simulink model "pid_model_selector_motorlibreria"  (R2019b)
settings: Solver=FixedStepAuto  StartTime=0  StopTime=0.02  FixedStep=1e-7  RelTol=1e-3
values from neighbouring files (symbols this model uses):
  duty_input_voltage_100 = 1    [pid_values_motorlibreria.m]    (also in pid_values_motorlibreria_OperationPointA.m; pid_values_motorlibreria_OperationPointB.m; pid_values_motorlibreria_OperationPointC.m)
  Kb = 0    [pid_values_motorlibreria.m]    (also in pid_values_motorlibreria_OperationPointA.m = 0.00333333333333; pid_values_motorlibreria_OperationPointB.m = 0.00333333333333; pid_values_motorlibreria_OperationPointC.m = 0.00333333333333)
  Kd = 0    [pid_values_motorlibreria.m]    (also in pid_values_motorlibreria_OperationPointA.m; pid_values_motorlibreria_OperationPointB.m; pid_values_motorlibreria_OperationPointC.m)
  Ki = 0    [pid_values_motorlibreria.m]    (also in pid_values_motorlibreria_OperationPointA.m = 300; pid_values_motorlibreria_OperationPointB.m = 300; pid_values_motorlibreria_OperationPointC.m = 300)
  Kp = 1    [pid_values_motorlibreria.m]    (also in pid_values_motorlibreria_OperationPointA.m = 10; pid_values_motorlibreria_OperationPointB.m = 10; pid_values_motorlibreria_OperationPointC.m = 10)
  max_speed = 9500    [pid_values_motorlibreria.m]    (also in pid_values_motorlibreria_OperationPointA.m; pid_values_motorlibreria_OperationPointB.m; pid_values_motorlibreria_OperationPointC.m)
  motor_load = 251.26    [pid_values_motorlibreria.m]    (also in pid_values_motorlibreria_OperationPointA.m = -251.26; pid_values_motorlibreria_OperationPointB.m = -167.8; pid_values_motorlibreria_OperationPointC.m = -100.5)
  out_max = 1    [pid_values_motorlibreria.m]    (also in pid_values_motorlibreria_OperationPointA.m; pid_values_motorlibreria_OperationPointB.m; pid_values_motorlibreria_OperationPointC.m)
  out_min = -1    [pid_values_motorlibreria.m]    (also in pid_values_motorlibreria_OperationPointA.m; pid_values_motorlibreria_OperationPointB.m; pid_values_motorlibreria_OperationPointC.m)
  rads2rpm = 60/2/pi    (= 9.54929658551)    [pid_values_motorlibreria_OperationPointA.m]    (also in pid_values_motorlibreria_OperationPointB.m; pid_values_motorlibreria_OperationPointC.m)
  rotor_inertia = 536    [pid_values_motorlibreria.m]    (also in pid_values_motorlibreria_OperationPointA.m; pid_values_motorlibreria_OperationPointB.m; pid_values_motorlibreria_OperationPointC.m)
  speed_command = 3800    [pid_values_motorlibreria_OperationPointA.m]    (also in pid_values_motorlibreria_OperationPointB.m = 5690; pid_values_motorlibreria_OperationPointC.m = 9500)
undefined symbols (not defined in the file or in its folder): sigbuilder_block
libraries: fl_lib x10, nesl_utility x7, powerlib_meascontrol x4, ee_lib x3
settings Model: Creator=B00417  LastModifiedBy=B00417
settings SolverCC: ZeroCrossAlgorithm=Adaptive  AlgebraicLoopSolver=LineSearch
settings DebuggingCC: IgnoredZcDiagnostic=none

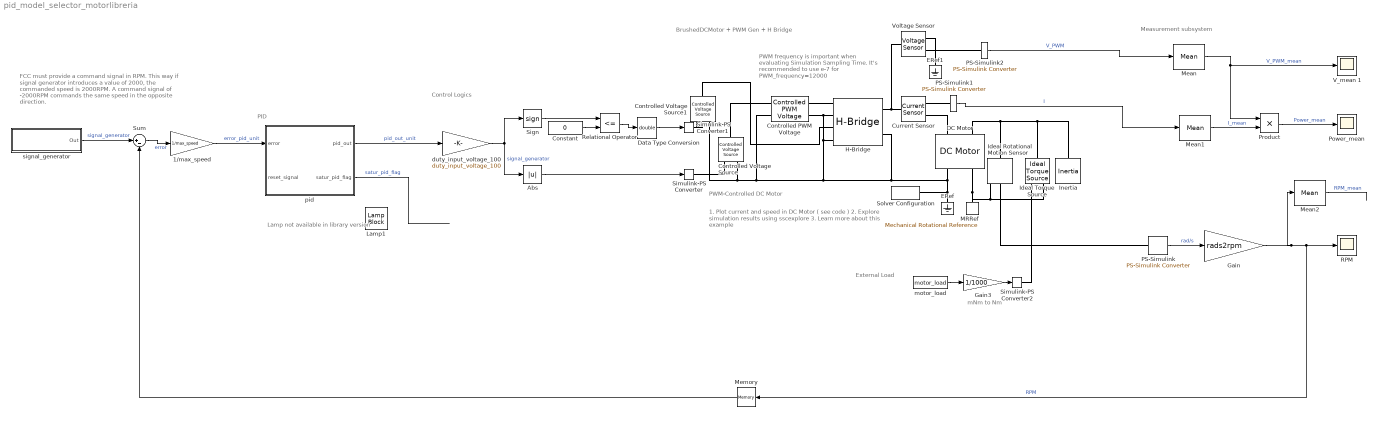
== system pid_model_selector_motorlibreria ==
  note: PWM frequency is important when evaluating Simulation Sampling Time.
      | It's recommended to use e-7 for PWM_frequency=12000
  note: External Load
  note: Control Logics
  note: FCC must provide a command signal in RPM. This way if signal generator introduces a value of 2000, the commanded speed is 2000RPM. A command signal of -2000RPM commands the same speed in the opposite direction.
  note: PID
  note: Lamp not available in library version
  note: Measurement subsystem
  note: BrushedDCMotor
      | + PWM Gen
      | + H Bridge
  note: mNm to Nm
  note: PWM-Controlled DC Motor
  note: 1. Plot current and speed in DC Motor ( see code )
      | 2. Explore simulation results using sscexplore
      | 3. Learn more about this example
  1/max_speed : Gain  Gain=1/max_speed
  Abs : Abs
  Constant : Constant  Value=0
  Controlled PWM Voltage : ee_lib/Integrated Circuits/Controlled PWM Voltage  F=PWM_frequency Hz  TD=PWM_delay s  pulse_width_offset=PWM_pulse_width_offset s  pulse_min=PWM_minimum_pulse_width s  Vmin=duty_input_voltage_0 V  Vmax=duty_input_voltage_100 V  Vm=V_duty_output V  pwm_or_av=1  event_type=1  sample_time=5e-6 s  u_min=0  u_max=1
      settings: SourceProductName=Simscape Electrical
  Controlled Voltage Source : fl_lib/Electrical/Electrical Sources/Controlled Voltage Source
  Controlled Voltage Source1 : fl_lib/Electrical/Electrical Sources/Controlled Voltage Source
  Current Sensor : fl_lib/Electrical/Electrical Sensors/Current Sensor
  DC Motor : ee_lib/Electromechanical/Brushed Motors/DC Motor  parameterization=2  Ra=3.38 Ohm  La=armature_inductance H  emf_or_torque=1  Kv=0.029 V/(rad/s)  Ki=6.876e-04 N*m/A  T_stall=stall_torque mN*m  w_max=no_load_speed rpm  w_rated=rated_speed rpm  P_rated=rated_load W  V_rated=rated_DC_V_supply V  J=rotor_inertia g*cm^2  lam_param=1  lam=rotor_damping N*m/(rad/s)  i_noload=728 mA  V_i_noload=20 V  speed0=0 rpm  alpha=3.93e-3 1/K  Tmeas=25 degC  thermal_mass=100 J/K  initial_temperature=25 degC
      settings: SourceProductName=Simscape Electrical
  Data Type Conversion : DataTypeConversion  OutMin=[0]  OutMax=[1]  OutDataTypeStr=double
  ERef : fl_lib/Electrical/Electrical Elements/Electrical Reference
  ERef1 : fl_lib/Electrical/Electrical Elements/Electrical Reference
  Gain : Gain  Gain=rads2rpm
  Gain3 : Gain  Gain=1/1000
  H-Bridge : ee_lib/Semiconductors & Converters/Converters/H-Bridge  supply_ports=ee.enum.supply_ports.hidesupply  Venable=V_enable V  Vmax=PWM_signal_amplitude V  Vreverse=REV_V V  Vbrake=BRK_V V  Vm=output_V V  pwm_or_av=ee.enum.pwm_or_av.pwm  regenerative_braking_mode=ee.enum.converters.regenerative_braking_mode.always_enabled  discontinuous=ee.enum.current_profile.continuous  freewheeling_mode=ee.enum.converters.freewheeling_mode.one_switch_one_diode  Ron=bridge_resistance Ohm  Don=diode_resistance Ohm  Goff=1e-6 S  Rload=3.38+0.1 Ohm  Lload=1e-5 H  F=4 kHz  thermal_mass=100 J/K  initial_temperature=298.15 K  Ron2=0.1 Ohm  Don2=0.05 Ohm  Tmeas=298.15 K  Tmeas2=398.15 K
      settings: SourceProductName=Simscape Electrical
  Ideal Rotational Motion Sensor : fl_lib/Mechanical/Mechanical Sensors/Ideal Rotational Motion Sensor  offset=0 deg
  Ideal Torque Source : fl_lib/Mechanical/Mechanical Sources/Ideal Torque Source
  Inertia : fl_lib/Mechanical/Rotational Elements/Inertia  inertia=motor_load_inertia kg*m^2  w_specify=off  w_priority=High  w=0 rad/s  w_nominal_specify=off  w_nominal_unit=rad/s  w_nominal_value=1  t_specify=off  t_priority=None  t=0 N*m  t_nominal_specify=off  t_nominal_unit=N*m  t_nominal_value=1
  Lamp1 : LampBlock
  MRRef : fl_lib/Mechanical/Rotational Elements/Mechanical Rotational Reference
  Mean : powerlib_meascontrol/Measurements/Mean  Freq=fundamental_frequency  Vinit=0  Ts=0
      settings: SourceProductName=Simscape Electrical
  Mean1 : powerlib_meascontrol/Measurements/Mean  Freq=fundamental_frequency  Vinit=0  Ts=0
      settings: SourceProductName=Simscape Electrical
  Mean2 : powerlib_meascontrol/Measurements/Mean  Freq=fundamental_frequency  Vinit=0  Ts=0
      settings: SourceProductName=Simscape Electrical
  Memory : Memory
  PS-Simulink : nesl_utility/PS-Simulink Converter  PhysicalDomain=network_engine_domain  SubClassName=ps_output  LeftPortType=input  RightPortType=output  PseudoPeriodic=off  Frequencies=[]  Unit=rpm  AffineConversion=off
  PS-Simulink1 : nesl_utility/PS-Simulink Converter  PhysicalDomain=network_engine_domain  SubClassName=ps_output  LeftPortType=input  RightPortType=output  PseudoPeriodic=off  Frequencies=[]  Unit=A  AffineConversion=off
  PS-Simulink2 : nesl_utility/PS-Simulink Converter  PhysicalDomain=network_engine_domain  SubClassName=ps_output  LeftPortType=input  RightPortType=output  PseudoPeriodic=off  Frequencies=[]  Unit=V  AffineConversion=off
  Power_mean : Scope
  Product : Product
  "RPM " : Scope
  Relational Operator : RelationalOperator  Operator=<=  OutDataTypeStr=boolean  RndMeth=Simplest
  Sign : Signum
  Simulink-PS Converter : nesl_utility/Simulink-PS Converter  PhysicalDomain=network_engine_domain  SubClassName=ps_input  LeftPortType=input  RightPortType=output  PseudoPeriodic=off  Frequencies=[]  NoiseDistribution=none  NoiseParameters=[]  Unit=1  AffineConversion=off  FilteringAndDerivatives=provide  SimscapeFilterOrder=1  InputFilterTimeConstant=0.001  UdotUserProvided=0
  Simulink-PS Converter1 : nesl_utility/Simulink-PS Converter  PhysicalDomain=network_engine_domain  SubClassName=ps_input  LeftPortType=input  RightPortType=output  PseudoPeriodic=off  Frequencies=[]  NoiseDistribution=none  NoiseParameters=[]  Unit=1  AffineConversion=off  FilteringAndDerivatives=provide  SimscapeFilterOrder=1  InputFilterTimeConstant=0.001  UdotUserProvided=0
  Simulink-PS Converter2 : nesl_utility/Simulink-PS Converter  PhysicalDomain=network_engine_domain  SubClassName=ps_input  LeftPortType=input  RightPortType=output  PseudoPeriodic=off  Frequencies=[]  NoiseDistribution=none  NoiseParameters=[]  Unit=1  AffineConversion=off  FilteringAndDerivatives=provide  SimscapeFilterOrder=1  InputFilterTimeConstant=0.001  UdotUserProvided=0
  Solver Configuration : nesl_utility/Solver Configuration  PhysicalDomain=network_engine_domain  SubClassName=solver  LeftPortType=input  RightPortType=generic  Tones=[]  Harmonics=[]  SimulateNoise=off  Profile=off  UseLocalSampling=off  EnableSwitchedLinearOptims=on  FrequencyDomain=off  UseCCode=off  RelTol=0.001  AbsTol=1e-06  MinStep=1e-09  ToWorkspace=off  RevertToSquareIcSolve=off  NumHomotopyIterations=100  PhasorMode=off  PhasorModeNumHarmonics=1  DoDC=off  ResidualTolerance=1e-9  UseLocalSolver=off  LocalSolverChoice=NE_BACKWARD_EULER_ADVANCER  LocalSolverSampleTime=1e-7  DoFixedCost=off  MaxNonlinIter=4  MaxModeIter=2  LinearAlgebra=auto  EquationFormulation=NE_TIME_EF  DelaysMemoryBudget=1024  AutomaticFiltering=on  FilteringTimeConstant=0.001  PartitionStorageMethod=AS_NEEDED  PartitionMemoryBudget=1024  PartitionMethod=FAST
  Sum : Sum  Inputs=|+-
  V_mean 1 : Scope
  Voltage Sensor : fl_lib/Electrical/Electrical Sensors/Voltage Sensor
  duty_input_voltage_100 : Gain  Gain=duty_input_voltage_100
  motor_load : Constant  Value=motor_load
  pid : Subsystem  mask{Kp=Kp, Ki=Ki, Kd=Kd, saturation_off=off, x_max=out_max, x_min=out_min, Ka=Kb}
      mask prompts: Kp "Kp Ganancia proporcional"; Ki "Ki Ganancia integral"; Kd "Kd Ganancia derivativa"; saturation_off "saturation off"; x_max "Salida máxima saturación"; x_min "salida minima satración"; Ka "Kb Ganancia Windup"
      mask DialogControl wind_up_container Prompt: saturation
      mask Display: disp("PID")
  "signal_generator " : Subsystem  mask{signal=Step, A=speed_command, f=10, Bias=0, Tstart=0, SlewRate=10000, SlewRate_Switch=off}
      mask prompts: A "Amplitude A"; f "Frequency f (Hz)"; Tstart "Start time for step Tstart (s)"; SlewRate "Maximum Slew Rate (1/s)"; SlewRate_Switch "On/Off"
      mask help:
      | Signal_generator
      |
      | Necesita:
      | Entender que es BIOS
      | Saw no funciona (Arreglar)
      |
      | Info:
      | Slew rate es el ratio de subida máximo que permite un generador, generalmente se mide en V/segundo. En este caso, un valor de 1 hace que la pendiente máxima sea 1.
      mask TypeOptions signal: Constant | Step | Sine | Step series | Saw | Builder
      mask Callback signal:
      | 1;
      | 2;
      | 3;
      | 4;
      | 5;
      mask Display: disp('signal_generator')
  wires:
  "signal_generator "/1(Out) -> Sum/1  "signal_generator"
  Sum/1 -> 1/max_speed/1  "error"
  1/max_speed/1 -> pid/1(error)  "error_pid_unit"
  pid/1(pid_out) -> duty_input_voltage_100/1  "pid_out_unit"
  pid/2(satur_pid_flag) -> ?  "satur_pid_flag"
  Mean1/1 -> Product/2  "I_mean"
  Mean/1 -> Product/1, V_mean 1/1  "V_PWM_mean"
  Constant/1 -> Relational Operator/2
  Sign/1 -> Relational Operator/1
  Relational Operator/1 -> Data Type Conversion/1
  PS-Simulink2/1 -> Mean/1  "V_PWM"
  PS-Simulink1/1 -> Mean1/1  "I"
  Abs/1 -> Simulink-PS Converter/1
  Product/1 -> Power_mean/1  "Power_mean"
  motor_load/1 -> Gain3/1
  PS-Simulink/1 -> Gain/1  "rad/s"
  Gain3/1 -> Simulink-PS Converter2/1
  Data Type Conversion/1 -> Simulink-PS Converter1/1
  duty_input_voltage_100/1 -> Abs/1, Sign/1  "signal_generator"
  Gain/1 -> Mean2/1, Memory/1, "RPM "/1  "RPM"
  Memory/1 -> Sum/2
  Mean2/1 -> ?  "RPM_mean"
  connections:
  H-Bridge/LConn2 -- Controlled PWM Voltage/RConn2 -- H-Bridge/RConn2 -- DC Motor/RConn1 -- Solver Configuration/RConn1 -- ERef/LConn1 -- Controlled Voltage Source1/RConn2 -- Controlled Voltage Source/RConn2 -- Controlled PWM Voltage/LConn2 -- H-Bridge/LConn4
  H-Bridge/RConn1 -- Voltage Sensor/LConn1 -- Current Sensor/LConn1
  MRRef/LConn1 -- Ideal Torque Source/RConn2 -- Ideal Rotational Motion Sensor/RConn1 -- DC Motor/RConn2
  Simulink-PS Converter/RConn1 -- Controlled Voltage Source/RConn1
  Current Sensor/RConn2 -- DC Motor/LConn1
  Simulink-PS Converter2/RConn1 -- Ideal Torque Source/RConn1
  Controlled Voltage Source1/LConn1 -- H-Bridge/LConn3
  Controlled Voltage Source/LConn1 -- Controlled PWM Voltage/LConn1
  Controlled PWM Voltage/RConn1 -- H-Bridge/LConn1
  Simulink-PS Converter1/RConn1 -- Controlled Voltage Source1/RConn1
  Current Sensor/RConn1 -- PS-Simulink1/LConn1
  Voltage Sensor/RConn1 -- PS-Simulink2/LConn1
  Ideal Rotational Motion Sensor/RConn2 -- PS-Simulink/LConn1
  DC Motor/LConn2 -- Ideal Rotational Motion Sensor/LConn1 -- Ideal Torque Source/LConn1 -- Inertia/LConn1
  Voltage Sensor/RConn2 -- ERef1/LConn1

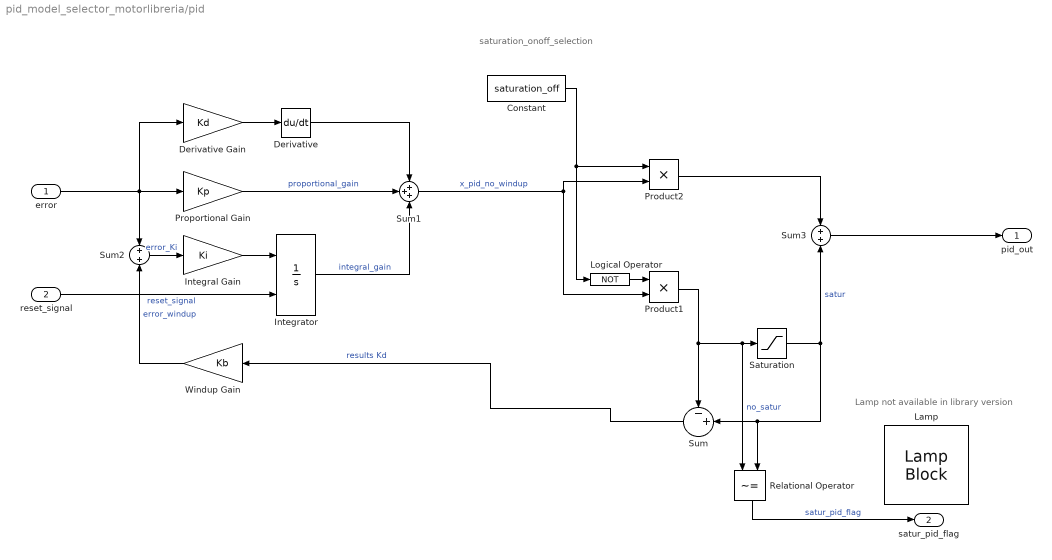
== system pid_model_selector_motorlibreria/pid ==
  note: Lamp not available in library version
  note: saturation_onoff_selection
  error : Inport
  reset_signal : Inport  Port=2
  Constant : Constant  Value=saturation_off
  Derivative : Derivative
  Derivative Gain : Gain  Gain=Kd
  Integral Gain : Gain  DisableCoverage=on  Gain=Ki
  Integrator : Integrator  ExternalReset=falling
  Lamp : LampBlock
  Logical Operator : Logic  Operator=NOT  AllPortsSameDT=off  OutDataTypeStr=boolean
  Product1 : Product
  Product2 : Product
  Proportional Gain : Gain  Gain=Kp
  Relational Operator : RelationalOperator  Operator=~=  OutDataTypeStr=boolean  RndMeth=Simplest
  Saturation : Saturate  UpperLimit=x_max  LowerLimit=x_min
  Sum : Sum  Inputs=-+|
  Sum1 : Sum  Inputs=+++
  Sum2 : Sum  Inputs=+|+
  Sum3 : Sum  Inputs=+|+
  Windup Gain : Gain  DisableCoverage=on  Gain=Kb
  pid_out : Outport
  satur_pid_flag : Outport  Port=2
  wires:
  Integrator/1 -> Sum1/3  "integral_gain"
  Integral Gain/1 -> Integrator/1
  error/1 -> Derivative Gain/1, Proportional Gain/1, Sum2/1
  Sum1/1 -> Product1/2, Product2/2  "x_pid_no_windup"
  Proportional Gain/1 -> Sum1/2  "proportional_gain"
  reset_signal/1 -> Integrator/2  "reset_signal"
  Saturation/1 -> Sum3/2, Relational Operator/2, Sum/2  "satur"
  Sum2/1 -> Integral Gain/1  "error_Ki"
  Sum/1 -> Windup Gain/1  "results Kd"
  Windup Gain/1 -> Sum2/2  "error_windup"
  Derivative Gain/1 -> Derivative/1
  Derivative/1 -> Sum1/1
  Relational Operator/1 -> satur_pid_flag/1  "satur_pid_flag"
  Sum3/1 -> pid_out/1
  Product2/1 -> Sum3/1
  Product1/1 -> Saturation/1, Relational Operator/1, Sum/1  "no_satur"
  Constant/1 -> Product2/1, Logical Operator/1
  Logical Operator/1 -> Product1/1

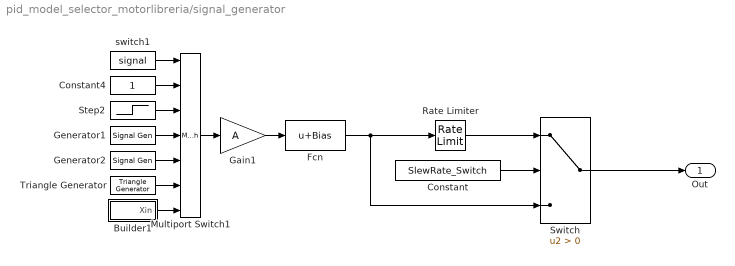
== system pid_model_selector_motorlibreria/signal_generator  ==
  Builder1 : Subsystem  Tag=STV Subsys  LoadFcn=sigbuilder_block('load');  StartFcn=sigbuilder_block('start');  StopFcn=sigbuilder_block('stop');  ClipboardFcn=sigbuilder_block('clipboard');  mask(Sigbuilder block){tuvar=[0:10]}
      mask help: Simulink:masks:SigbuilderBlock_MD
      mask init:
      | if ~strcmp(get_param(bdroot(gcbh),'SimulationStatus'),'stopped') tuvar = sigbuilder_block('maskInit'); end
      settings: CopyFcn=sigbuilder_block('copy');  DeleteFcn=sigbuilder_block('delete');  ModelCloseFcn=sigbuilder_block('modelClose');  PreSaveFcn=sigbuilder_block('preSave');  PauseFcn=sigbuilder_block('pause')  ContinueFcn=sigbuilder_block('continue')  NameChangeFcn=sigbuilder_block('namechange');  OpenFcn=sigbuilder_block('open',[-14.25 -14.25 1213.5 669 ]);  CloseFcn=sigbuilder_block('close');
      mask Display: plot(0, 0, 100, 100,[2, 2, 32, 32, 2], [68, 8, 8, 68, 68],[32, 2], [38, 38], [32, 19, 2],[53, 60, 44], [32, 17, 17, 2],[16, 16, 31, 31]);txt = getActiveGroup(gcbh);text(2, 100, txt,'verticalAlignment', 'top');
  Constant : Constant  Value=SlewRate_Switch
  Constant4 : Constant
  Fcn : Fcn  Expr=u+Bias
  Gain1 : Gain  Gain=A
  Generator1 : SignalGenerator  Frequency=f
      mask Display: disp('Sine')
  Generator2 : SignalGenerator  WaveForm=square  Frequency=f
      mask Display: disp('Square')
  Multiport Switch1 : MultiPortSwitch  Inputs=6
  Rate Limiter : RateLimiter  RisingSlewLimit=SlewRate  FallingSlewLimit=-SlewRate  SampleTimeMode=inherited
  Step2 : Step  Time=Tstart  SampleTime=0
  Switch : Switch  Criteria=u2 > Threshold
  Triangle Generator : powerlib_meascontrol/Pulse & Signal Generators/Triangle Generator  Freq=f  Phase=90  Ts=0
      settings: SourceProductName=Simscape Electrical
  switch1 : Constant  Value=signal
  Out : Outport
  wires:
  Rate Limiter/1 -> Switch/1
  Constant/1 -> Switch/2
  Fcn/1 -> Rate Limiter/1, Switch/3
  Triangle Generator/1 -> Multiport Switch1/6
  Builder1/1(Xin) -> Multiport Switch1/7
  Generator2/1 -> Multiport Switch1/5
  switch1/1 -> Multiport Switch1/1
  Gain1/1 -> Fcn/1
  Multiport Switch1/1 -> Gain1/1
  Step2/1 -> Multiport Switch1/3
  Generator1/1 -> Multiport Switch1/4
  Constant4/1 -> Multiport Switch1/2
  Switch/1 -> Out/1

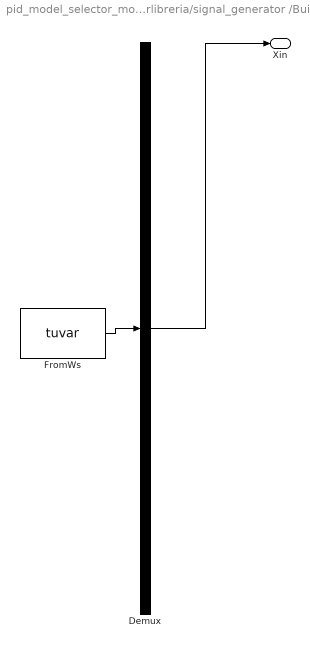
== system pid_model_selector_motorlibreria/signal_generator /Builder1 ==
  Demux : Demux  Tag=STV Demux  Outputs=1
  FromWs : FromWorkspace  Tag=STV FromWs  VariableName=tuvar  SampleTime=0
      SigBuilderData=|
      | common.afterFinalStr = 'Extrapolate'
      | common.sampleTime = 0
      | dataSet.timeRange = [0 10]
      | dataSet.name = 'Control'
      | sbobj.Groups.Name = 'Control'
      | sbobj.Groups.Signals.Name = 'Xin'
      | sbobj.Groups.Signals.XData = [0 1.99 1.99 10]
      | sbobj.Groups.Signals.YData = [1 1 2.002 2]
  Xin : Outport  Tag=STV Outport
  wires:
  Demux/1 -> Xin/1
  FromWs/1 -> Demux/1
